simulink model "Tutorial3"  (R2022a)
settings: Solver=FixedStepAuto  StartTime=0.0  StopTime=10.0  FixedStep=1e-3  RelTol=1e-3  EnableMultiTasking=on
libraries: frdmk64flib x5, etargetslib x2
settings Model: ExtModeTrigDuration=5  Creator=bmile  LastModifiedBy=bmile
settings OptimizationCC: EnhancedBackFolding=on  PassReuseOutputArgsAs=Individual arguments  ZeroExternalMemoryAtStartup=off  ZeroInternalMemoryAtStartup=off  MaxStackSize=64  OptimizeBlockOrder=speed  DifferentSizesBufferReuse=on  OptimizationCustomize=off  EfficientTunableParamExpr=on
settings DebuggingCC: ParameterTunabilityLossMsg=error
settings HardwareCC: ProdBitPerPointer=32  ProdBitPerSizeT=32  ProdBitPerPtrDiffT=32  ProdLargestAtomicInteger=Long  ProdLargestAtomicFloat=Double  ProdWordSize=32  ProdHWDeviceType=ARM Compatible->ARM Cortex
settings SFSimCC: MATLABDynamicMemAlloc=off
settings RTWCC: SystemTargetFile=ert.tlc  HardwareBoard=NXP FRDM-K64F  TLCOptions="-aInlineSetEventsForThisBaseRateFcn=TLC_FALSE -aSuppressMultiTaskScheduler=TLC_FALSE  -aRateBasedStepFcn=0"  TemplateMakefile=ert_default_tmf  Toolchain=GNU Tools for ARM Embedded Processors
settings CodeAppCC: ForceParamTrailComments=on  IgnoreCustomStorageClasses=off  OperatorAnnotations=on  SimulinkDataObjDesc=on  SFDataObjDesc=on  InsertBlockDesc=on
settings ERTTargetCC: ExtModeTransport=4  ExtModeMexFile=sendToCommService

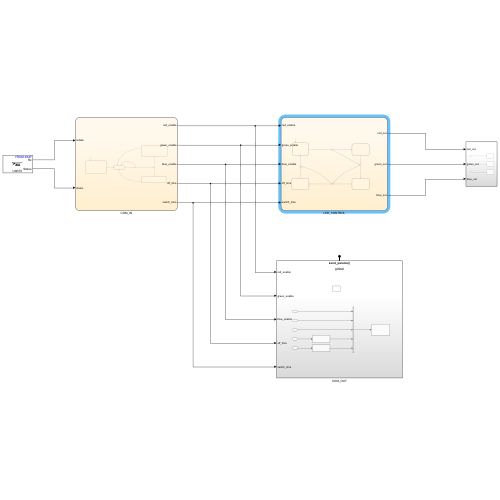
[thumbnail: Simulink's stored preview of the top-level diagram]
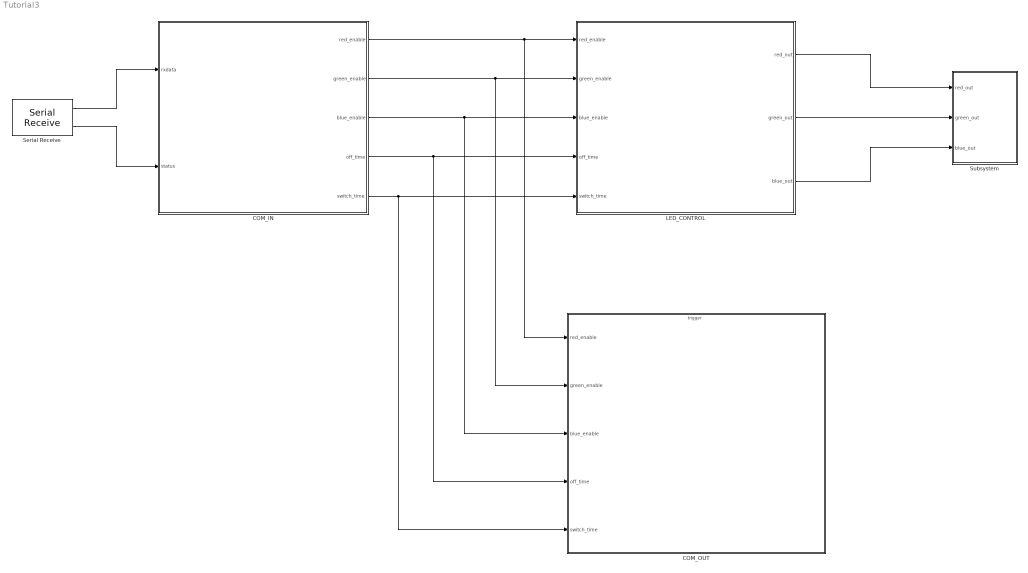
== system Tutorial3 ==
  COM_IN : Stateflow chart  TreatAsAtomicUnit=on
      settings: PortSchema="{\"entries\":[{\"content\":{\"sides\":[{\"content\":{\"connectorIds\":[\"In1\",\"In2\"]},\"type\":\"ConnectorPlacement.EquallySpacedRectSide\",\"uuid\":\"81a31a14-91e3-4f35-a4fd-cbefb3419df2\"},{\"content\":{\"connectorIds\":[\"Out4\",\"Out3\",\"Out1\",\"Out2\",\"Out5\"],\"side\":\"RIGHT\"},\"type\":\"ConnectorPlacement.EquallySpacedRectSide\",\"uuid\":\"035cc0cb-2e4b-401d-a886-d384cf234001\"},{\"content\":{\"connectorIds\":[],\"side\":\"TOP\"},\"type\":\"ConnectorPlacement.EquallySpacedRectSide\",\"uuid\":\"ccb3e4fa-663a-44e3-94d5-8113de75fb4f\"}]},\"type\":\"ConnectorPlacement.EquallySpacedConnector\",\"uuid\":\"e37e0753-821b-457a-99c5-a86105689923\"}],\"packageUris\":[\"http://schema.mathworks.com/mf0/Connector/R2020b\"],\"version\":\"1.0\"}"
  COM_OUT : Subsystem
  LED_CONTROL : Stateflow chart  TreatAsAtomicUnit=on
      settings: PortSchema="{\"entries\":[{\"content\":{\"sides\":[{\"content\":{\"connectorIds\":[\"In1\",\"In2\",\"In3\",\"In4\",\"In5\"]},\"type\":\"ConnectorPlacement.EquallySpacedRectSide\",\"uuid\":\"3978b6dd-a69b-41f5-930e-5049bd6743bc\"},{\"content\":{\"connectorIds\":[\"Out2\",\"Out3\",\"Out1\"],\"side\":\"RIGHT\"},\"type\":\"ConnectorPlacement.EquallySpacedRectSide\",\"uuid\":\"ad05e6e2-3523-4aad-8e69-d4c735154bf8\"},{\"content\":{\"connectorIds\":[],\"side\":\"TOP\"},\"type\":\"ConnectorPlacement.EquallySpacedRectSide\",\"uuid\":\"43e2de5b-60ac-4a27-8f26-73f9d49ab55c\"}]},\"type\":\"ConnectorPlacement.EquallySpacedConnector\",\"uuid\":\"26ef1e99-3fde-43ff-8c5e-2fd65b8a8ad3\"}],\"packageUris\":[\"http://schema.mathworks.com/mf0/Connector/R2020b\"],\"version\":\"1.0\"}"
  Serial Receive : frdmk64flib/Serial Receive  SCIModule=0  Baudrate=uint32(9600)  Parity=None  StopBits=1  HardwareFlowControl=None  ByteOrder=LittleEndian  DataType=uint8  DataLength=11  BlockingMode=off  OutputStatus=on  SampleTime=-1
  Subsystem : Subsystem
  wires:
  COM_IN/4(red_enable) -> COM_OUT/1(red_enable), LED_CONTROL/1(red_enable)
  COM_IN/3(green_enable) -> COM_OUT/2(green_enable), LED_CONTROL/2(green_enable)
  COM_IN/1(blue_enable) -> COM_OUT/3(blue_enable), LED_CONTROL/3(blue_enable)
  COM_IN/2(off_time) -> COM_OUT/4(off_time), LED_CONTROL/4(off_time)
  COM_IN/5(switch_time) -> COM_OUT/5(switch_time), LED_CONTROL/5(switch_time)
  LED_CONTROL/2(red_out) -> Subsystem/1(red_out)
  LED_CONTROL/3(green_out) -> Subsystem/2(green_out)
  LED_CONTROL/1(blue_out) -> Subsystem/3(blue_out)
  Serial Receive/1 -> COM_IN/1(rxdata)
  Serial Receive/2 -> COM_IN/2(status)

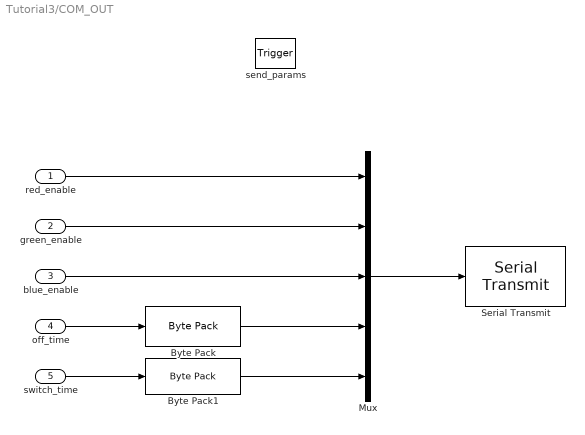
== system Tutorial3/COM_OUT ==
  red_enable : Inport
  green_enable : Inport  Port=2
  blue_enable : Inport  Port=3
  off_time : Inport  Port=4
  switch_time : Inport  Port=5
  send_params : TriggerPort  TriggerType=function-call  IsSimulinkFunction=on  FunctionName=send_params  VariantControl=Variant  PortDimensions=1
  Byte Pack : etargetslib/Byte Pack  datatypes={'single'}  byteAlign=1
  Byte Pack1 : etargetslib/Byte Pack  datatypes={'uint16'}  byteAlign=1
  Mux : Mux  Inputs=5
  Serial Transmit : frdmk64flib/Serial Transmit  SCIModule=0  Baudrate=uint32(9600)  Parity=None  StopBits=1  HardwareFlowControl=None  ByteOrder=LittleEndian  BlockingMode=on  OutputStatus=off
  wires:
  off_time/1 -> Byte Pack/1
  switch_time/1 -> Byte Pack1/1
  red_enable/1 -> Mux/1
  green_enable/1 -> Mux/2
  blue_enable/1 -> Mux/3
  Byte Pack/1 -> Mux/4
  Byte Pack1/1 -> Mux/5
  Mux/1 -> Serial Transmit/1

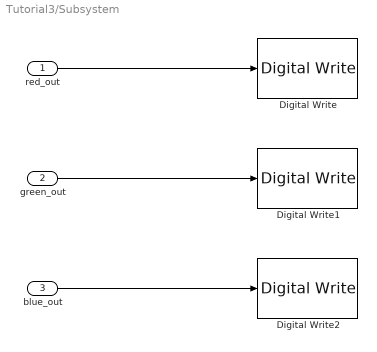
== system Tutorial3/Subsystem ==
  red_out : Inport
  green_out : Inport  Port=2
  blue_out : Inport  Port=3
  Digital Write : frdmk64flib/Digital Write  Whichpin=RED_LED
  Digital Write1 : frdmk64flib/Digital Write  Whichpin=GREEN_LED
  Digital Write2 : frdmk64flib/Digital Write  Whichpin=BLUE_LED
  wires:
  blue_out/1 -> Digital Write2/1
  green_out/1 -> Digital Write1/1
  red_out/1 -> Digital Write/1

== stateflow chart Tutorial3/LED_CONTROL ==
  state OFF
    entry:
    red_out = 0;
    green_out = 0;
    blue_out = 0;
  state RED_ON
    entry:
    red_out = 1;
    green_out = 0;
    blue_out = 0;
  state BLUE_ON
    entry:
    red_out = 0;
    green_out = 0;
    blue_out = 1;
  state GREEN_ON
    entry:
    red_out = 0;
    green_out = 1;
    blue_out = 0;
  (default) -> OFF
  OFF -> (junction 8) : after(off_time, sec)
  (junction 8) -> RED_ON [order 1] : [red_enable == 1]
  (junction 8) -> (junction 14) [order 2]
  (junction 16) -> OFF
  RED_ON -> (junction 14) : after(switch_time,msec)
  (junction 14) -> (junction 15) [order 2]
  (junction 14) -> GREEN_ON [order 1] : [green_enable == 1]
  (junction 15) -> (junction 16) [order 2]
  BLUE_ON -> (junction 16) : after(switch_time, msec)
  (junction 15) -> BLUE_ON [order 1] : [blue_enable == 1]
  GREEN_ON -> (junction 15) : after(switch_time, msec)
  data: red_enable input; green_enable input; blue_enable input; off_time input; switch_time input; blue_out output; red_out output; green_out output

== stateflow chart Tutorial3/COM_IN ==
  settings: executeAtInitialization=1
  state SET_PARAM
    entry:
    red_enable = rxdata(3);
    green_enable = rxdata(4);
    blue_enable = rxdata(5);
    off_time = typecast(rxdata(6:9), 'single');
    switch_time = typecast(rxdata(10:11), 'uint16');
  state INITIAL
    %Set the initial values of parameters
    entry:
    red_enable = 1;
    green_enable = 1;
    blue_enable = 0;
    off_time = 0.5; % in seconds
    switch_time = 200; % in ms
  state STANDBY
    %Waits for COM
  state ECHO_PARAM
    entry:
    send_params();
  SET_PARAM -> STANDBY
  (junction 15) -> SET_PARAM [order 1] : [rxdata(2) == 55]
  (default) -> INITIAL
  (junction 12) -> STANDBY [order 2]
  INITIAL -> STANDBY
  STANDBY -> (junction 12) : [status == 0]
  (junction 12) -> (junction 15) [order 1] : [rxdata(1) == 22]
  (junction 15) -> ECHO_PARAM [order 2] : [rxdata(2) == 22]
  ECHO_PARAM -> STANDBY
  data: rxdata input uint8; status input uint8; blue_enable output uint8; off_time output single; green_enable output uint8; red_enable output uint8; switch_time output uint16
